simulink model "Hibrido"  (R2021b)
settings: Solver=VariableStepAuto  StartTime=0.0  StopTime=50  RelTol=1e-3
settings Model: Creator=duart  LastModifiedBy=duart

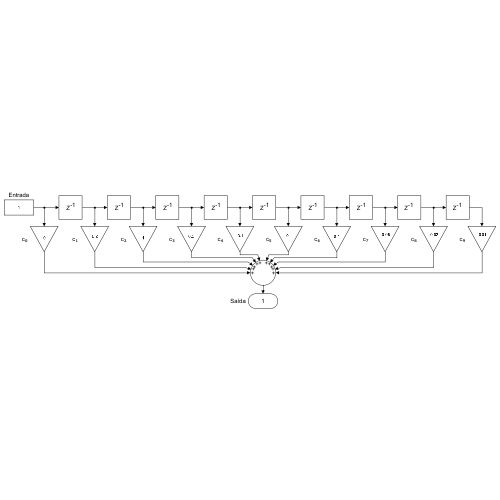
[thumbnail: Simulink's stored preview of the top-level diagram]
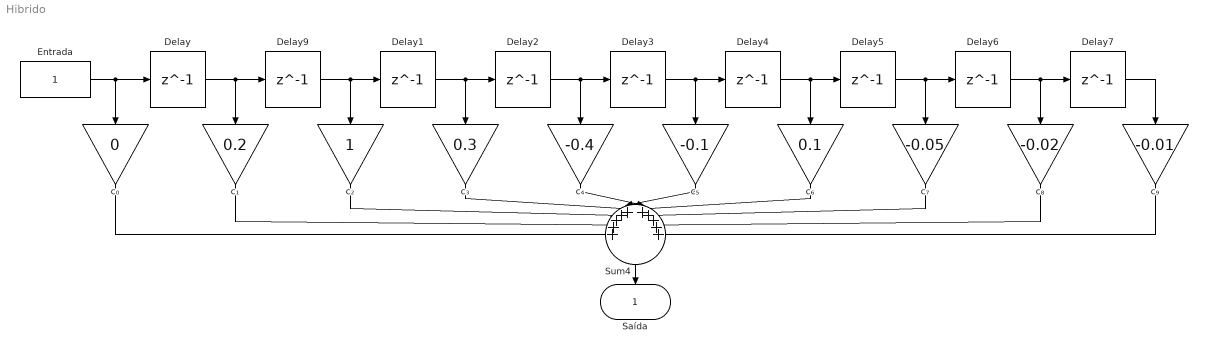
== system Hibrido ==
  Delay{,1..7,9} (9 alike) : Delay  DelayLength=1  InitialCondition=0
  Entrada : Constant
  Sum4 : Sum  Inputs=+++++|+++++
  c₀ : Gain  Gain=0
  c₁ : Gain  Gain=0.2
  c₂ : Gain
  c₃ : Gain  Gain=0.3
  c₄ : Gain  Gain=-0.4
  c₅ : Gain  Gain=-0.1
  c₆ : Gain  Gain=0.1
  c₇ : Gain  Gain=-0.05
  c₈ : Gain  Gain=-0.02
  c₉ : Gain  Gain=-0.01
  Saída : Outport
  wires:
  Entrada/1 -> Delay/1, c₀/1
  Delay2/1 -> Delay3/1, c₄/1
  Delay1/1 -> Delay2/1, c₃/1
  Delay9/1 -> Delay1/1, c₂/1
  Delay/1 -> Delay9/1, c₁/1
  c₉/1 -> Sum4/10
  c₈/1 -> Sum4/9
  c₇/1 -> Sum4/8
  c₆/1 -> Sum4/7
  c₅/1 -> Sum4/6
  c₄/1 -> Sum4/5
  c₃/1 -> Sum4/4
  c₂/1 -> Sum4/3
  c₁/1 -> Sum4/2
  c₀/1 -> Sum4/1
  Sum4/1 -> Saída/1
  Delay3/1 -> Delay4/1, c₅/1
  Delay4/1 -> c₆/1, Delay5/1
  Delay5/1 -> Delay6/1, c₇/1
  Delay6/1 -> Delay7/1, c₈/1
  Delay7/1 -> c₉/1
